simulink library "Lib_Controls"  (Simulink 8.3)
settings: Solver=ode45  StartTime=0.0  StopTime=10.0  RelTol=1e-3
undefined symbols (not defined in the file): avgACCactiveTime, LearnGain
settings Model: Creator=swami  LastModifiedBy=swami

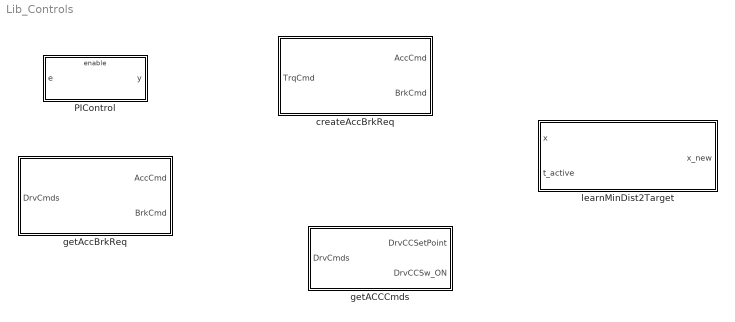
== system Lib_Controls ==
  PIControl : Subsystem  mask{Kp=0, Ki=0}
  createAccBrkReq : Subsystem
  getACCCmds : Subsystem
  getAccBrkReq : Subsystem
  learnMinDist2Target : Subsystem

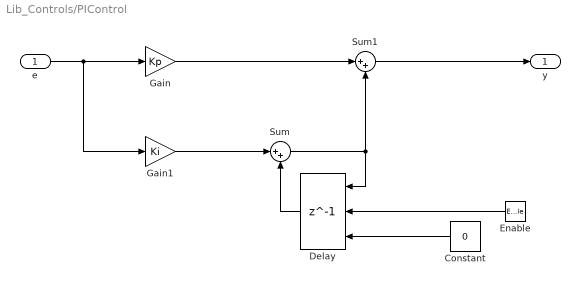
== system Lib_Controls/PIControl ==
  e : Inport
  Enable : EnablePort  ShowOutputPort=on
  Constant : Constant  Value=0
  Delay : Delay  DelayLength=1  InitialConditionSource=Input port  InitialCondition=0  ExternalReset=Rising
      settings: InputPortMap=u0,r5,p4
  Gain : Gain  Gain=Kp
  Gain1 : Gain  Gain=Ki
  Sum : Sum  Inputs=|++
  Sum1 : Sum  Inputs=|++
  y : Outport
  wires:
  e/1 -> Gain1/1, Gain/1
  Gain1/1 -> Sum/1
  Sum/1 -> Sum1/2, Delay/1
  Delay/1 -> Sum/2
  Gain/1 -> Sum1/1
  Enable/1 -> Delay/2
  Constant/1 -> Delay/3
  Sum1/1 -> y/1

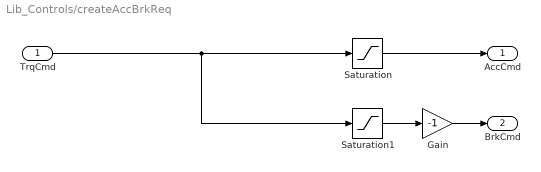
== system Lib_Controls/createAccBrkReq ==
  TrqCmd : Inport
  Gain : Gain  Gain=-1
  Saturation : Saturate  UpperLimit=inf  LowerLimit=0
  Saturation1 : Saturate  UpperLimit=0  LowerLimit=-inf
  AccCmd : Outport
  BrkCmd : Outport  Port=2
  wires:
  Saturation1/1 -> Gain/1
  Saturation/1 -> AccCmd/1
  TrqCmd/1 -> Saturation/1, Saturation1/1
  Gain/1 -> BrkCmd/1

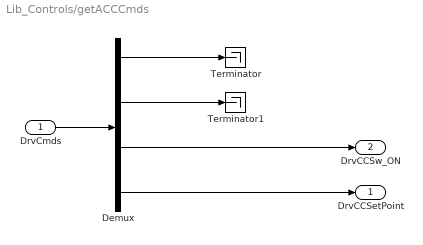
== system Lib_Controls/getACCCmds ==
  DrvCmds : Inport  OutDataTypeStr=double  PortDimensions=4
  Demux : Demux
  Terminator : Terminator
  Terminator1 : Terminator
  DrvCCSetPoint : Outport
  DrvCCSw_ON : Outport  Port=2
  wires:
  DrvCmds/1 -> Demux/1
  Demux/3 -> DrvCCSw_ON/1
  Demux/4 -> DrvCCSetPoint/1
  Demux/1 -> Terminator/1
  Demux/2 -> Terminator1/1

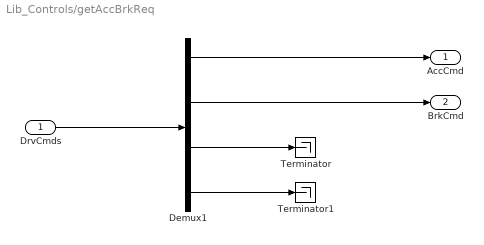
== system Lib_Controls/getAccBrkReq ==
  DrvCmds : Inport
  Demux1 : Demux
  Terminator : Terminator
  Terminator1 : Terminator
  AccCmd : Outport
  BrkCmd : Outport  Port=2
  wires:
  DrvCmds/1 -> Demux1/1
  Demux1/3 -> Terminator/1
  Demux1/4 -> Terminator1/1
  Demux1/1 -> AccCmd/1
  Demux1/2 -> BrkCmd/1

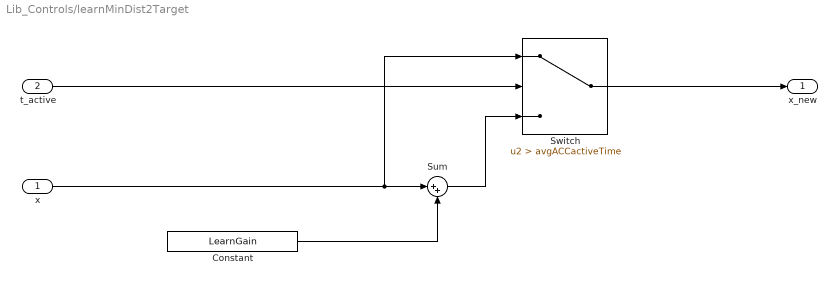
== system Lib_Controls/learnMinDist2Target ==
  x : Inport  OutDataTypeStr=double  PortDimensions=1
  t_active : Inport  Port=2  OutDataTypeStr=double  PortDimensions=1
  Constant : Constant  Value=LearnGain
  Sum : Sum  Inputs=|++
  Switch : Switch  Criteria=u2 > Threshold  Threshold=avgACCactiveTime
  x_new : Outport
  wires:
  Sum/1 -> Switch/3
  Switch/1 -> x_new/1
  Constant/1 -> Sum/2
  x/1 -> Switch/1, Sum/1
  t_active/1 -> Switch/2
